simulink model "assg_2"  (R2021a)
settings: Solver=VariableStepAuto  StartTime=0.0  StopTime=10.0  RelTol=1e-3
values from neighbouring files (symbols this model uses):
  A = [0,0,1,0;0,0,0,1;0,g*m_p/m_c,-d1/m_c,-d2/(L*m_c);0,g*(m_c+m_p)/(L*m_c),-d1/(L*m_c),-d2*(m_c+m_p)/((L^2)*m_c*m_p)]    [assgn_2.m]
  B = [0;0;1/m_c;1/(L*m_c)]    [assgn_2.m]
  c = [0,1,0,0]    [assgn_2.m]
  D = [0]    [assgn_2.m]
settings Model: Creator=Aastik  LastModifiedBy=Aastik

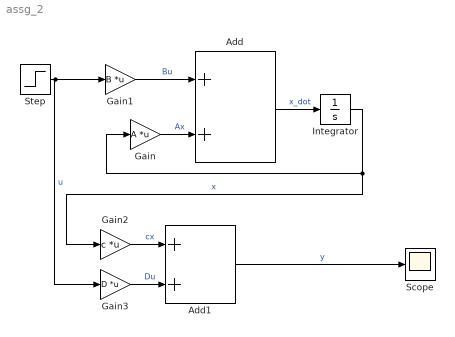
== system assg_2 ==
  Add : Sum
  Add1 : Sum
  Gain : Gain  Gain=A  Multiplication=Matrix(K*u)
  Gain1 : Gain  Gain=B  Multiplication=Matrix(K*u)
  Gain2 : Gain  Gain=c  Multiplication=Matrix(K*u)
  Gain3 : Gain  Gain=D  Multiplication=Matrix(K*u)
  Integrator : Integrator
  Scope : Scope
  Step : Step  Before=100  SampleTime=0
  wires:
  Add/1 -> Integrator/1  "x_dot"
  Integrator/1 -> Gain2/1, Gain/1  "x"
  Step/1 -> Gain3/1, Gain1/1  "u"
  Gain1/1 -> Add/1  "Bu"
  Gain/1 -> Add/2  "Ax"
  Gain2/1 -> Add1/1  "cx"
  Gain3/1 -> Add1/2  "Du"
  Add1/1 -> Scope/1  "y"
